simulink model "baseline1"  (R2022b)
settings: Solver=ode4  StartTime=0.0  StopTime=200  FixedStep=1e-3  RelTol=1e-3
undefined symbols (not defined in the file or in its folder): A_do, B_do, c_uf, do_w, f_b, f_max, f_min, F_TOT_MAX, Fz_min, g, G_do, Gamma_mix, Ixx, Iyy, Izz, K_eta, K_omega, K_w, Ka1, Ka2, Ka3, Kgamma, Knu, Kp1, Kp2, Kp3, L, l_axis, l_gain, m, m_p, n_state_axis, p2_bias_acc, p2_h3_s0, p2_ic_do, p2_ic_eso, p2_ic_pos, p2_ic_vel, p2_nd_pos, p2_prm, p2_prm_h3, p2_prm_m3, p2_prm_n6, p2_prm_w, p2_seed_acc, p2_seed_gyro, p2_seed_pos, p2_tau_m, p2_trim_do, p2_trim_eso, p2_trim_ff_v, p2_Ts_att, p2_Ts_pos, p2_var_acc, p2_var_gyro, p2_var_pos, payload_amp, payload_inj_on, payload_K_ratio, payload_model ... (+18)
(part 2 of 3)

== matlab function baseline1/Disturbances/Payload_Pendulum/pend_out ==
  data: xp input; d_mf output; a_uav input; m_p input; L input; g input; payload_z_on input
function d_mf = payload_pendulum_output(xp, a_uav, m_p, L, g, payload_z_on)
%#codegen
%PAYLOAD_PENDULUM_OUTPUT  Luc cap truyen len UAV = nhieu tai d_mf.
%
%  Paste noi dung file nay vao mot khoi MATLAB Function RIENG.
%  Tach roi khoi payload_pendulum_derivative theo dung kieu ma model dang
%  dung cho DO (do_derivative / do_output) va ESO.
%
%  Luc cang cap, moi truc:
%     T = m_p*( g*cos(th) + L*thdot^2 + a*sin(th) )
%  Phan luc ngang len UAV:
%     d = T*sin(th)
%
%  KHOP VOI BASELINE.  Trong translational_dynamics:
%     m*nu_dot = F - m*g*e3 + d_mf + d_lf
%  nen d_mf la LUC, don vi N, he QUAN TINH.  Dung het - khong chia khoi
%  luong, khong doi frame, khong doi dau.
%
%  ----------------------------------------------------------------------
%  THE VERTICAL COMPONENT (payload_z_on) - Part 3.5 (TEST_PLAN_PROMPT.md)
%  ----------------------------------------------------------------------
%  The tether pulls the UAV DOWN with force T*cos(th). At hover (th ~ 0),
%  T ~ m_p*g, so this pull is the payload's static weight - and it belongs
%  in the trim, not out of it: translational_dynamics.m's own equilibrium
%  (nu_dot = 0) gives F_act(3) = m*g - d_mf(3), so d_mf(3) = -T*cos(th)
%  makes the controller command F_act(3) = m*g + T ~ (m + m_p)*g at hover -
%  exactly the physical thrust margin table above, and exactly what
%  Checkpoint 3.5 measures.
%
%  An EARLIER version of this block computed d_z = m_p*g - T*cos(th_eff)
%  instead - subtracting the payload's own weight back out, so d_z ~ 0 at
%  hover and the trim point stayed IDENTICAL to m*g with no payload at all.
%  That was deliberate at the time (docs/devlog/AUDIT.md item 11 names it a
%  documented limitation, not an oversight): payload_z_on was reserved for a
%  future ablation and had never been turned on for any locked result, so
%  nothing published depended on its old behaviour. Checkpoint 3.5 is that
%  future ablation, and it explicitly requires the opposite: the payload's
%  weight DOES have to move the trim point, or "total thrust = (m + m_p)*g"
%  cannot be measured at all. Removing the +m_p*g cancellation term is the
%  whole fix.
%
%  payload_z_on = 0  (DEFAULT, unchanged - Stage 2.1's own bit-exact gate)
%     d_mf(3) = 0, identical to the original baseline (d_mf was horizontal
%     only). Only ONE thing differs between payload_model = 0 and 1: the
%     horizontal disturbance waveform. One experiment, one variable.
%  payload_z_on = 1
%     Adds the FULL vertical reaction, constant term included. Hover, no
%     wind: position stable, no saturation, total thrust = (m + m_p)*g
%     within 1% (Checkpoint 3.5) - not the near-zero-mean oscillation the
%     earlier version produced.

d_mf = zeros(3,1);

th_x = xp(1);  thd_x = xp(2);
th_y = xp(3);  thd_y = xp(4);

T_x = m_p*( g*cos(th_x) + L*thd_x^2 + a_uav(1)*sin(th_x) );
T_y = m_p*( g*cos(th_y) + L*thd_y^2 + a_uav(2)*sin(th_y) );

d_mf(1) = T_x*sin(th_x);
d_mf(2) = T_y*sin(th_y);

if payload_z_on > 0.5
    % Combined swing angle, used to project the tether tension onto z.
    th_eff  = sqrt(th_x^2 + th_y^2);
    T_eff   = m_p*( g*cos(th_eff) + L*(thd_x^2 + thd_y^2) );
    % Full reaction, including its constant (trim-shifting) part - see the
    % header. NOT m_p*g - T_eff*cos(th_eff): that cancelled the constant
    % term back out, which is exactly what Checkpoint 3.5 says must not
    % happen anymore.
    d_mf(3) = -T_eff*cos(th_eff);
end
end

== matlab function baseline1/Position_Observers/Payload_Predictor/pred_fcn ==
  data: gamma input; dmf_hat_p output; nu input; z input; l_gain input; do_w input; n_state_axis input; tau_pred input
function dmf_hat_p = payload_predictor(gamma, nu, z, l_gain, do_w, n_state_axis, tau_pred)
%#codegen
%PAYLOAD_PREDICTOR  Physical predictor for the payload disturbance: dmf_hat(t + tau).
%
%  Inputs
%     gamma, nu     : UAV position / velocity, inertial frame
%     z             : disturbance observer (DO) state, FLAT across all 3 axes
%     l_gain        : the DO's l gain (same as the DO_Out block)
%     do_w          : each exosystem block's frequency, FLAT across all 3
%                     axes, in the SAME order build_do_matrices.m used to
%                     build z (axis 1 in full, then axis 2, then axis 3)
%     n_state_axis  : 3x1, the number of STATES (not frequencies) each
%                     axis owns within z/xi_hat - Part 3.3 (TEST_PLAN_PROMPT.md)
%     tau_pred      : prediction horizon, s
%  Output
%     dmf_hat_p : the payload disturbance estimate AT TIME t + tau_pred, 3x1, N
%
%  ----------------------------------------------------------------------
%  PART 3.3: WHY n_state_axis WAS ADDED INSTEAD OF MAKING do_w A CELL
%  ----------------------------------------------------------------------
%  build/build_do_matrices.m's new form takes do_w_axis, a CELL {wx,wy,wz}
%  - but this is a %#codegen Simulink MATLAB Function block, and every
%  signal crossing a Simulink wire needs a FIXED SIZE at compile time;
%  Simulink cannot carry a cell type across a signal line. do_w here STAYS
%  a FLAT vector (exactly as before), just no longer IMPLICITLY split into
%  three equal shares - n_state_axis(i) says EXACTLY how many STATES (not
%  how many do_w entries) belong to axis i, and this function works out
%  how many do_w entries that is by accumulating block sizes (1 for DC, 2
%  for a harmonic) until that target is reached - the same logic
%  build_do_matrices.m uses to turn do_w_axis{i} into states, run in
%  reverse here.
%
%  With n_state_axis = [n_as;n_as;n_as] (all three axes equal, the
%  original case) and do_w in the OLD order, the loop below consumes
%  exactly n_as states per axis, identical to the old behaviour - which is
%  why Checkpoint 3.3's bit-exact gate (circle) needs no special-case branch.
%
%  ----------------------------------------------------------------------
%  DERIVATION (unchanged)
%  ----------------------------------------------------------------------
%  DO gia thiet nhieu tai sinh boi mot exosystem tuyen tinh, pt. (6):
%       xi_dot = A*xi,      d_mf = B*xi
%  Neu gia thiet do dung thi trang thai tuong lai biet duoc chinh xac:
%       xi(t + tau) = e^{A*tau} * xi(t)
%  va uoc luong hien tai la xi_hat = z + l*[gamma; nu]  (pt. 11a). Nen:
%       dmf_hat_p = B * e^{A*tau} * xi_hat
%
%  A la khoi cheo cac khoi 2x2 [0 w; -w 0], moi khoi mot tan so. e^{A*tau}
%  vi vay la mot phep QUAY, va MOI KHOI QUAY MOT GOC KHAC NHAU: khoi o tan so
%  w quay goc w*tau.
%       e^{A_k*tau} = [ cos(w_k*tau)   sin(w_k*tau);
%                      -sin(w_k*tau)   cos(w_k*tau) ]
%  Khong can expm - hai ham luong giac cho moi khoi.
%
%  B lay thanh phan LE cua moi khoi va CONG chung lai (d_mf cua mot truc la
%  tong dong gop cua cac hoa), nen chi can hang thu nhat cua moi phep quay:
%       dmf_hat_p(i) = sum_k [ cos(w_k*tau)*xi(le_k) + sin(w_k*tau)*xi(chan_k) ]
%
%  ----------------------------------------------------------------------
%  STATE ORDER - must match build_do_matrices
%  ----------------------------------------------------------------------
%  By AXIS first, then by FREQUENCY (in the order do_w_axis{i} lists them):
%       [axis1_freq1(1 or 2), axis1_freq2(...), axis2_freq1(...), ...]
%  With n_state_axis equal across axes and do_w in the old order, this
%  reduces to exactly the original 6/9/... state layout.
%
%  BLOCKS OF DIFFERENT SIZES, NOW ALSO ACROSS AXES (new - Part 3.3):
%  frequency 0 is the ONE-DIMENSIONAL DC mode, 1 state (§0.68 - 97.8% of
%  the payload channel's model error is a constant force); any other
%  frequency takes 2. The original code ASSUMED all 3 axes had the SAME
%  state count (numel(z) == 3*n_as); this one no longer does -
%  n_state_axis states it separately per axis.
%
%  ----------------------------------------------------------------------
%  TAU_PRED (unchanged)
%  ----------------------------------------------------------------------
%  Bang do tre HIEU DUNG tren duong luc, DO DUOC chu khong tinh ra: quet tau
%  o nhanh sin cho thay diem triet tieu (RMS_y = RMS_x) o tau = 140 ms.
%  Mo hinh chi tinh vong tu the bac hai cho 93 ms, nen ~47 ms den tu phan mo
%  hinh do khong co (phi tuyen thrust_attitude_ref, quan sat tu the, C(eta)).
%  Xem docs/AUDIT.md muc E.
%
%  ----------------------------------------------------------------------
%  GIOI HAN - PHAI GHI TRONG PAPER (khong doi)
%  ----------------------------------------------------------------------
%  Phep quay lay ca thanh phan CHAN cua exosystem vao dau ra. Thanh phan do
%  khong duoc quan sat truc tiep (B chi lay thanh phan le) nen sai so uoc
%  luong cua no lon hon, va bo du doan khuech dai no len theo sin(w*tau).
%  Do duoc: residual cua nhanh sin tang tu 0.0024 N (tau = 0) len 0.0118 N
%  (tau = 140 ms), voi mot vach moi hien ra dung o tan so sigma.
%  Do la mot gioi han tren THAT cho viec tang tau, khong phai loi cai dat.

dmf_hat_p = zeros(3,1);

xi_hat = z + l_gain*[gamma; nu];        % pt. (11a), giong DO_Out

% *** LOCK DIMENSIONS, per-axis version. ***
% If n_state_axis(i) does not match z's real state count, this fails
% SILENTLY in exactly the way the original warning described: the block
% keeps running, still outputs three plausible-looking numbers, just
% picking up the wrong axis's states. The assert below is the only guard.
assert(numel(n_state_axis) == 3, ...
    'payload_predictor: n_state_axis must have 3 elements.');
assert(sum(n_state_axis) == numel(z), ...
    ['payload_predictor: n_state_axis sums to %d, which does not match ' ...
     'z''s state count (%d). The Constant block feeding n_state_axis or ' ...
     'do_w is pointing at the wrong variable - re-run build_payload_predictor.'], ...
    sum(n_state_axis), numel(z));

n_w = numel(do_w);
b  = 0;   % state pointer (into z / xi_hat)
kw = 0;   % frequency pointer (into do_w)
for i = 1:3
    acc = 0;
    consumed = 0;
    while consumed < n_state_axis(i)
        kw = kw + 1;
        assert(kw <= n_w, ...
            'payload_predictor: ran out of do_w before axis %d had enough states.', i);
        w = do_w(kw);
        if w == 0
            % e^{0*tau} = 1: a constant predicts itself. This is why this
            % mode can never "predict wrong" - it only needs to be ESTIMATED.
            acc = acc + xi_hat(b+1);
            b = b + 1;
            consumed = consumed + 1;
        else
            c = cos(w*tau_pred);
            s = sin(w*tau_pred);
            acc = acc + c*xi_hat(b+1) + s*xi_hat(b+2);
            b = b + 2;
            consumed = consumed + 2;
        end
    end
    dmf_hat_p(i) = acc;
end
end

== matlab function baseline1/Position_Observers/IM_Est_Online/IM_Estimator ==
  data: vx input; w_hat_x output; vy input; t input; trust_x output; w_hat_y output; trust_y output; w_all_x output; mag_all_x output; w_all_y output; mag_all_y output
function [w_hat_x, trust_x, w_hat_y, trust_y, ...
          w_all_x, mag_all_x, w_all_y, mag_all_y] = im_est_estimator(vx, vy, t)
%#codegen
%IM_EST_ESTIMATOR  Online AR(2n) RLS + eig-based root-finding + Nyquist/
%  DC exclusion + per-slot nearest-neighbour assignment + trust gate +
%  coasting (docs/REGISTER_C.md sec 4.29/4.35/4.47). A codegen MATLAB
%  Function (Stateflow/EML) block - the SAME proven block type
%  Position_Observers/DO_12 (do_derivative) and Payload_Predictor
%  (payload_predictor) already use in this repo, not the legacy
%  Interpreted MATLAB Function block (multi-port support for that one
%  could not be verified without a MATLAB session to test against).
%  persistent state is standard, documented MATLAB Coder/Embedded
%  MATLAB practice. Every array here is FIXED SIZE (order=8 slots,
%  NaN-padded past the real count) - no dynamically-growing arrays, no
%  logical-index compaction, no nested structs - specifically to avoid
%  the variable-size codegen uncertainty that motivated (and then
%  un-motivated, sec 4.47) earlier design changes. Runs at fs=1Hz,
%  inherited from its input's sample time (the upstream Zero-Order
%  Hold in production; a From Workspace block at checkpoint 1.5).
%
%  Mirrors core/im_est_rls.m's own RLS update EXACTLY - same phi
%  convention (phi = -[x(k-1)..x(k-order)]), same lambda/order -
%  incrementally rather than in a batch loop, specifically so
%  checkpoint 1.5's 1e-9 rad/s agreement against that already-trusted
%  offline computation is a real regression test, not a coincidence.
%
%  Root-finding uses eig() of the companion matrix, not roots() -
%  roots() itself builds this same companion matrix internally and
%  calls eig() on it, so the values are identical by construction.
%
%  Untrusted slots (docs/REGISTER_C.md sec 4.29/4.35): |z|>=0.97 AND
%  <5% drift over the trailing 10 s AND t>=15s (a global floor, not a
%  per-slot "time since first trusted"). w_hat reports the 0.3 rad/s
%  placeholder for an untrusted slot - the internal tracking state is
%  NOT overwritten to the placeholder, so a slowly-converging slot
%  keeps its own continuity rather than being reset every untrusted
%  tick.
%
%  w_all_x/mag_all_x/w_all_y/mag_all_y (DIAGNOSTIC ONLY, sec 4.47
%  checkpoint 1.5): the raw ORDER=8 root set, BEFORE Nyquist/DC_GUARD
%  filtering or merging - directly comparable, element set for element
%  set (sort before comparing), to core/im_est_rls.m's own
%  R.roots(k,:) on identical input. Left unwired in the production
%  embedding - kept in this one file rather than forked into a second
%  copy, so the tested code and the deployed code never drift apart.

N_PAIRS = 4;
ORDER = 8;                      % 2*N_PAIRS, written as a literal for
                                 % codegen's fixed-size inference
LAM = 0.99;
NYQ_CUT = 0.9*pi;                % 0.9*Nyquist at DT_D = 1.0 s
DC_GUARD = 0.02;
DOMEGA_MIN = 0.05;
PLACEHOLDER = 0.3;
DRIFT_WIN = 10;
DRIFT_TOL = 0.05;
T_FLOOR = 15;

persistent theta_x theta_y P_x P_y buf_x buf_y n_seen_x n_seen_y
persistent slot_w_x slot_w_y slot_hist_x slot_hist_y

if isempty(n_seen_x)
    theta_x = zeros(ORDER,1); theta_y = zeros(ORDER,1);
    P_x = eye(ORDER)*1e3;     P_y = eye(ORDER)*1e3;
    buf_x = zeros(1,ORDER);   buf_y = zeros(1,ORDER);
    n_seen_x = 0;             n_seen_y = 0;
    slot_w_x = PLACEHOLDER*ones(1,N_PAIRS);
    slot_w_y = PLACEHOLDER*ones(1,N_PAIRS);
    slot_hist_x = PLACEHOLDER*ones(DRIFT_WIN,N_PAIRS);
    slot_hist_y = PLACEHOLDER*ones(DRIFT_WIN,N_PAIRS);
end

[theta_x, P_x, buf_x, n_seen_x, slot_w_x, slot_hist_x, w_hat_x, trust_x, w_all_x, mag_all_x] = ...
    tick_axis(theta_x, P_x, buf_x, n_seen_x, slot_w_x, slot_hist_x, vx, t, ...
    ORDER, N_PAIRS, LAM, NYQ_CUT, DC_GUARD, DOMEGA_MIN, PLACEHOLDER, DRIFT_TOL, T_FLOOR);
[theta_y, P_y, buf_y, n_seen_y, slot_w_y, slot_hist_y, w_hat_y, trust_y, w_all_y, mag_all_y] = ...
    tick_axis(theta_y, P_y, buf_y, n_seen_y, slot_w_y, slot_hist_y, vy, t, ...
    ORDER, N_PAIRS, LAM, NYQ_CUT, DC_GUARD, DOMEGA_MIN, PLACEHOLDER, DRIFT_TOL, T_FLOOR);
end

%% =====================================================================
function [theta, P, buf, n_seen, slot_w, slot_hist, w_hat, trust, w_all, mag_all] = ...
    tick_axis(theta, P, buf, n_seen, slot_w, slot_hist, v, t, order, n_pairs, ...
    lam, nyq_cut, dc_guard, domega_min, placeholder, drift_tol, t_floor)

% ---- RLS update (core/im_est_rls.m's own equations, incremental) ----
n_seen = n_seen + 1;
if n_seen > order
    phi   = -buf(:);
    e     = v - phi.'*theta;
    Pphi  = P*phi;
    denom = lam + phi.'*Pphi;
    Kk    = Pphi/denom;
    theta = theta + Kk*e;
    P     = (P - Kk*(Pphi.'))/lam;
end
buf = [v, buf(1:end-1)];

% ---- root-finding: companion matrix, eig() ----
c = theta(:).';
C = zeros(order,order);
C(1,:) = -c;
C(2:order,1:order-1) = eye(order-1);
r = eig(C);

w_all = abs(angle(r)).';          % 1 x order, DT_D = 1.0 s
mag_all = abs(r).';               % 1 x order

% ---- Nyquist/DC_GUARD exclusion + close-frequency merge, FIXED SIZE
% (order slots, NaN = not present) - no dynamically-growing arrays ----
w_cand = nan(1,order); m_cand = nan(1,order);
keep = (w_all <= nyq_cut) & (w_all > dc_guard);
w_tmp = w_all; w_tmp(~keep) = NaN;
m_tmp = mag_all; m_tmp(~keep) = NaN;
[w_tmp_sorted, ord] = sort(w_tmp);           % NaNs sort to the end
m_tmp_sorted = m_tmp(ord);
n_cand = 0;
for i = 1:order
    if isnan(w_tmp_sorted(i)), continue; end
    if n_cand > 0 && (w_tmp_sorted(i) - w_cand(n_cand) < domega_min)
        if m_tmp_sorted(i) > m_cand(n_cand)
            w_cand(n_cand) = w_tmp_sorted(i);
            m_cand(n_cand) = m_tmp_sorted(i);
        end
    else
        n_cand = n_cand + 1;
        w_cand(n_cand) = w_tmp_sorted(i);
        m_cand(n_cand) = m_tmp_sorted(i);
    end
end

% ---- greedy nearest-neighbour slot assignment (sec 4.29 item 4a);
% unmatched slots COAST - slot_w stays at its previous value. Fixed
% size throughout: n_pairs slots, order candidate cells (only the
% first n_cand are ever valid, the rest are NaN and never selected). ----
assigned = false(1,n_pairs);
mag_assigned = zeros(1,n_pairs);
avail = ~isnan(w_cand);
for pass = 1:n_pairs
    bestSlot = 0; bestCand = 0; bestDist = Inf;
    for s = 1:n_pairs
        if assigned(s), continue; end
        for k = 1:order
            if ~avail(k), continue; end
            d = abs(w_cand(k) - slot_w(s));
            if d < bestDist
                bestDist = d; bestSlot = s; bestCand = k;
            end
        end
    end
    if bestSlot == 0, break; end
    slot_w(bestSlot) = w_cand(bestCand);
    mag_assigned(bestSlot) = m_cand(bestCand);
    assigned(bestSlot) = true;
    avail(bestCand) = false;
end

slot_hist = [slot_hist(2:end,:); slot_w];

trust = false(1,n_pairs);
for s = 1:n_pairs
    h  = slot_hist(:,s);
    mh = mean(h);
    drift = (max(h)-min(h)) / max(mh, eps);
    trust(s) = assigned(s) && (mag_assigned(s) >= 0.97) && ...
               (drift < drift_tol) && (t >= t_floor);
end

w_hat = slot_w;
w_hat(~trust) = placeholder;
end

== matlab function baseline1/Position_Observers/IM_Est_Online/IM_Rebuild ==
  data: w_hat_x input; A_do output; trust_x input; w_hat_y input; trust_y input; wn_p input; sigma_z input; l_axis input; strict input; B_do output; l_gain output; G_do output; fallback output; reason output
function [A_do, B_do, l_gain, G_do, fallback, reason] = ...
    im_est_do_rebuild(w_hat_x, trust_x, w_hat_y, trust_y, wn_p, sigma_z, l_axis, strict)
%#codegen
%IM_EST_DO_REBUILD  Online IM = {0, w_hat_k, wn_p} internal-model
%  matrix rebuild (docs/REGISTER_C.md sec 4.29/4.35/4.46/4.47) - a
%  codegen MATLAB Function (Stateflow/EML) block, the SAME proven
%  block type as im_est_estimator.m and do_derivative/
%  payload_predictor, not build_do_matrices.m called directly:
%  build_do_matrices.m's cell-array/varargin dispatch is not verified
%  codegen-safe, and this function's do_w_axis STRUCTURE never varies
%  (always DC + 4 harmonics + wn_p on x/y, the unchanged {0,sigma_z}
%  on z - n_state = 25, fixed) - only the FREQUENCY VALUES at each
%  slot change - so a direct, fixed-index construction is used
%  instead, with build_do_matrices.m's own stability check (eig(A_cl)
%  < 0) replicated exactly. The CONSTRUCTION-EQUIVALENCE checkpoint
%  (sec 4.47) - forcing every slot to the exact-frequency reference's
%  own values and comparing against build_do_matrices's OWN output
%  bit for bit - exists specifically to catch a construction error
%  here, so drift is not asserted away, it is tested for.
%
%  State order (sec 4.46's own fixed layout, matching
%  build_do_matrices.m's "by axis first, then by frequency" rule with
%  the harmonics in slot order 1-4, then wn_p):
%    x: [1]=DC [2 3]=h1 [4 5]=h2 [6 7]=h3 [8 9]=h4 [10 11]=wn_p
%    y: [12]=DC [13 14]=h1 [15 16]=h2 [17 18]=h3 [19 20]=h4 [21 22]=wn_p
%    z: [23]=DC [24 25]=sigma_z
%
%  DECOUPLING (sec 4.47 item 3, the refinement to sec 4.29/4.35's
%  placeholder-only design): an untrusted harmonic slot (trust_x/y(k)
%  false) still occupies its 2 states (fixed size, sec 4.47's own
%  registered reasoning) but gets l_gain=0 for both AND is excluded
%  from B_do - completely inert, not merely mistuned. DC and wn_p are
%  never coasted/untrusted, so decoupling only ever applies to the 4
%  harmonic slots per axis.
%
%  FALLBACK (sec 4.46 item 1): candidate frequencies within
%  DOMEGA_MIN=0.05 rad/s of each other (checked among the axis's own
%  4 harmonics + wn_p - a defensive check on the REBUILD input, in
%  addition to im_est_estimator.m's own pre-assignment merge, sec
%  4.47's own note) OR a resulting UNSTABLE Acl -> HOLD the previous
%  A_do/B_do/l_gain (persistent, fixed-size - no Memory-block feedback
%  needed, same reasoning as im_est_estimator.m's own state) and
%  report fallback=true, reason (1=dup, 2=unstable). strict=true skips
%  the hold and errors immediately instead - for checkpoint-building
%  only, never a production/scored run (sec 4.46 item 1c).

N = 25;
DOMEGA_MIN = 0.05;
M_UAV = 1.121;

persistent A_prev B_prev L_prev initialized
if isempty(initialized)
    A_prev = zeros(N,N);
    B_prev = zeros(3,N);
    L_prev = zeros(N,6);
    initialized = true;
end

G_do = (1/M_UAV)*[zeros(3,3); eye(3)];

% ---- defensive dup check: each axis's own 4 harmonics + wn_p ----
% Only TRUSTED harmonics (+ wn_p, always trusted) can collide in a way
% that matters: a decoupled/untrusted slot is excluded from B_do and
% l_gain, so its frequency value never enters Acl's own observable
% dynamics - two untrusted slots sharing the SAME placeholder (as every
% slot does before any is trusted, during warmup) is not a real
% duplicate in the sense build_do_matrices.m's own assertion guards
% against, and must not spuriously trigger a fallback.
tx = [trust_x(1) trust_x(2) trust_x(3) trust_x(4) true];
dup = false;
fx = [w_hat_x(1) w_hat_x(2) w_hat_x(3) w_hat_x(4) wn_p];
for i = 1:5
    for j = i+1:5
        if tx(i) && tx(j) && abs(fx(i)-fx(j)) < DOMEGA_MIN, dup = true; end
    end
end
ty = [trust_y(1) trust_y(2) trust_y(3) trust_y(4) true];
fy = [w_hat_y(1) w_hat_y(2) w_hat_y(3) w_hat_y(4) wn_p];
for i = 1:5
    for j = i+1:5
        if ty(i) && ty(j) && abs(fy(i)-fy(j)) < DOMEGA_MIN, dup = true; end
    end
end

if dup && strict
    error('im_est_do_rebuild:dup', 'candidate frequencies within DOMEGA_MIN of each other (strict mode).');
end

A_new = zeros(N,N);
B_new = zeros(3,N);
L_new = zeros(N,6);

% ---- x axis: states 1..11 ----
A_new(1,1) = 0;  B_new(1,1) = 1;  L_new(1,4) = l_axis(1);
[A_new, B_new, L_new] = put_harm(A_new, B_new, L_new, 2, w_hat_x(1), l_axis(1), 1, trust_x(1));
[A_new, B_new, L_new] = put_harm(A_new, B_new, L_new, 4, w_hat_x(2), l_axis(1), 1, trust_x(2));
[A_new, B_new, L_new] = put_harm(A_new, B_new, L_new, 6, w_hat_x(3), l_axis(1), 1, trust_x(3));
[A_new, B_new, L_new] = put_harm(A_new, B_new, L_new, 8, w_hat_x(4), l_axis(1), 1, trust_x(4));
[A_new, B_new, L_new] = put_harm(A_new, B_new, L_new, 10, wn_p, l_axis(1), 1, true);

% ---- y axis: states 12..22 ----
A_new(12,12) = 0;  B_new(2,12) = 1;  L_new(12,5) = l_axis(2);
[A_new, B_new, L_new] = put_harm(A_new, B_new, L_new, 13, w_hat_y(1), l_axis(2), 2, trust_y(1));
[A_new, B_new, L_new] = put_harm(A_new, B_new, L_new, 15, w_hat_y(2), l_axis(2), 2, trust_y(2));
[A_new, B_new, L_new] = put_harm(A_new, B_new, L_new, 17, w_hat_y(3), l_axis(2), 2, trust_y(3));
[A_new, B_new, L_new] = put_harm(A_new, B_new, L_new, 19, w_hat_y(4), l_axis(2), 2, trust_y(4));
[A_new, B_new, L_new] = put_harm(A_new, B_new, L_new, 21, wn_p, l_axis(2), 2, true);

% ---- z axis: states 23..25 (unchanged {0, sigma_z} - never estimated) ----
A_new(23,23) = 0;  B_new(3,23) = 1;  L_new(23,6) = l_axis(3);
[A_new, B_new, L_new] = put_harm(A_new, B_new, L_new, 24, sigma_z, l_axis(3), 3, true);

% ---- stability check on the ACTIVE subsystem only ----
% A decoupled harmonic block still carries its own [0 w;-w 0] open-loop
% dynamics in A_new (by design - sec 4.47 item 3: the state exists and
% evolves, just isolated), whose eigenvalues sit exactly on the
% imaginary axis (Re=0) - marginally stable, not Re<0. Checking eig()
% of the FULL Acl would fail this test whenever ANY slot is untrusted,
% including the entire warmup period before t>=15s, which defeats the
% design (constant spurious fallback). Since a decoupled block is
% provably block-diagonal (B_new/L_new are both zero for it - no
% coupling in or out), its own marginal eigenvalues are harmless and
% irrelevant to whether the ACTIVE subsystem is stable. A_check patches
% each decoupled block's diagonal to a trivially-stable dummy (-I),
% fixed-index (no variable-size extraction needed) - it changes nothing
% about the ACTUAL A_do returned below, only what stability is
% evaluated against.
A_check = A_new;
A_check = patch_if_untrusted(A_check, 2,  trust_x(1));
A_check = patch_if_untrusted(A_check, 4,  trust_x(2));
A_check = patch_if_untrusted(A_check, 6,  trust_x(3));
A_check = patch_if_untrusted(A_check, 8,  trust_x(4));
A_check = patch_if_untrusted(A_check, 13, trust_y(1));
A_check = patch_if_untrusted(A_check, 15, trust_y(2));
A_check = patch_if_untrusted(A_check, 17, trust_y(3));
A_check = patch_if_untrusted(A_check, 19, trust_y(4));

Acl = A_check - L_new*G_do*B_new;
ev = eig(Acl);
stable = max(real(ev)) < 0;

if (~stable) && strict
    error('im_est_do_rebuild:unstable', 'Acl not stable with the current w_hat (strict mode).');
end

if dup || ~stable
    A_do = A_prev; B_do = B_prev; l_gain = L_prev;
    fallback = true;
    if dup, reason = 1; else, reason = 2; end
else
    A_do = A_new; B_do = B_new; l_gain = L_new;
    A_prev = A_new; B_prev = B_new; L_prev = L_new;
    fallback = false;
    reason = 0;
end
end

%% =====================================================================
function [A, B, L] = put_harm(A, B, L, idx1, w, lg, axis_col, trust)
%PUT_HARM  Place one 2-state harmonic block at states idx1,idx1+1 -
%  build_do_matrices.m's own [0 w;-w 0] / B_do(i,b+1)=1 / l_gain
%  pattern, fixed-index. trust=false -> decoupled (sec 4.47 item 3):
%  l_gain stays 0 for both states, B stays 0 - the state still exists
%  (fixed size) but contributes to and is corrected by nothing.
idx2 = idx1 + 1;
A(idx1,idx1) = 0;  A(idx1,idx2) = w;
A(idx2,idx1) = -w; A(idx2,idx2) = 0;
if trust
    B(axis_col, idx1) = 1;
    L(idx1, 3+axis_col) = lg;
    L(idx2, 3+axis_col) = lg;
end
end

%% =====================================================================
function A = patch_if_untrusted(A, idx1, trust)
%PATCH_IF_UNTRUSTED  For the stability check only (sec 4.47's own
%  reasoning, see the caller): a decoupled block's marginal (Re=0)
%  open-loop eigenvalues are harmless (B/l_gain are already zero for
%  it, so it cannot destabilize anything, block-diagonal) but would
%  otherwise fail max(real(eig(.)))<0 spuriously. Overwrite ONLY the
%  stability-check copy's diagonal block to a trivially-stable dummy.
if ~trust
    idx2 = idx1 + 1;
    A(idx1,idx1) = -1; A(idx1,idx2) = 0;
    A(idx2,idx1) = 0;  A(idx2,idx2) = -1;
end
end

== matlab function baseline1/P2/P2_Core/P2/P2_Trans ==
  data: x input double size=[12 1]; dx output double size=[12 1]; f_act input double size=1; eta input double size=[3 1]; w input double size=[3 1]; prm input double size=[8 1]; gam output double size=[3 1]; nu output double size=[3 1]; a_Q output double size=[3 1]; d_mf output double size=[3 1]; d_lf output double size=[3 1]; mon output double size=[5 1]
function [dx, gam, nu, a_Q, d_mf, d_lf, mon] = p2_trans(x, f_act, eta, w, prm)
%#codegen
%P2_TRANS  MATLAB Function block P2/P2_Core/P2/P2_Trans (GD2b, plant_model = 1).
%
%  Translational dynamics of the UAV + 3-D rigid-cable pendulum of plant P2. The
%  equations are NOT written here: this block calls core/plant_p2_free.m, the same
%  code verified offline by verification/verify_plant_p2.m (GD2a, 41/41).
%
%  In   x      12x1 state [x_Q; v_Q; q; omega] (Integrator P2_x, IC p2_x0)
%       f_act  total thrust AFTER the motor lag [N] (Gamma_mix * f, row 1)
%       eta    TRUE Euler angles (tag eta, Int_eta)
%       w      3x1 true wind [m/s]; the vertical component is dropped here (spec sec 5)
%       prm    [m_Q; m_L; L; g; zeta_s; K; K_w; U_ref]   (p2_prm, core/p2_setup.m)
%  Out  dx     12x1 state derivative
%       gam, nu, a_Q   true position, velocity, acceleration of the UAV
%       d_mf   T q - F_d  (cable force on the UAV, for logging)
%       d_lf   F_wQ       (wind force on the body, for logging)
%       mon    [T; slack; ||q|-1|; |omega.q|; theta]  (REGISTER_P2 sec 0.4 flags)

% Output sizes declared first (as every v1 block does, e.g. xp_dot = zeros(4,1)):
% the block sits in a loop with Integrator P2_x, and Simulink must know the output
% sizes before it knows the input sizes (GD2b, second build attempt).
dx   = zeros(12, 1);
gam  = zeros(3, 1);
nu   = zeros(3, 1);
a_Q  = zeros(3, 1);
d_mf = zeros(3, 1);
d_lf = zeros(3, 1);
mon  = zeros(5, 1);

P = struct('mode', 'free', 'g', prm(4), 'm_Q', prm(1), 'm_L', prm(2), 'L', prm(3), ...
           'zeta_s', prm(5), 'K', prm(6), 'K_w', prm(7), 'U_ref', prm(8));
F = force_from_attitude(f_act, eta);
[dx, o] = plant_p2_free(x, F, [w(1); w(2); 0], P);
gam  = x(1:3);
nu   = x(4:6);
a_Q  = dx(4:6);
d_mf = o.d_mf;
d_lf = o.d_lf;
qh   = x(7:9) / norm(x(7:9));
mon  = [o.T; double(o.slack); o.qnorm_err; o.wq; acos(max(min(-qh(3), 1), -1))];
end

== matlab function baseline1/P2/P2_Core/P2/P2_WindHat ==
  data: w input double size=[3 1]; dlf_hat output double size=[3 1]; nu_c input double size=[3 1]; prm_w input double size=[2 1]
function dlf_hat = p2_wind_force_hat(w, nu_c, prm_w)
%#codegen
%P2_WIND_FORCE_HAT  MATLAB Function block P2/P2_Core/P2/P2_WindHat (GD2b, plant_model = 1).
%
%  The controller's wind-force model on P2 (REGISTER_P2 sec 0.3): quadratic, the same
%  form as the plant's body drag, NOMINAL parameters, relative velocity w - v_Q with
%  the controller's own MEASURED velocity nu_c:
%     dlf_hat = (K_w/U_ref) |w - nu_c| (w - nu_c)
%  w is the SELECTED wind (sensor / PI-MoE / oracle, as WSEL); vertical component dropped.
%  prm_w = [K_w; U_ref]. Replaces K_w*w (WM_Kw / WP_Kw / WO_Kw) only when plant_model = 1.

dlf_hat = zeros(3, 1);          % output size declared first, as every v1 block does
r = [w(1); w(2); 0] - nu_c;
dlf_hat = (prm_w(1) / prm_w(2)) * norm(r) * r;
end

== matlab function baseline1/P2/P2_Core/P2/P2_N6 ==
  data: s input double size=[4 1]; s_next output double size=[4 1]; w_meas input double size=[3 1]; w_sig input double size=[3 1]; vQ input double size=[3 1]; dmf_do input double size=[3 1]; gate input double size=1; prm input double size=[17 1]; delta output double size=[3 1]; mon output double size=[5 1]
function [s_next, delta, mon] = p2_n6_term(s, w_meas, w_sig, vQ, dmf_do, gate, prm)
%#codegen
%P2_N6_TERM  MATLAB Function block P2/P2_Core/P2/P2_N6 (REGISTER_P2 sec 15.4, 18.2; N6).
%
%  Wind -> payload term added to the controller's payload channel (active only when
%  p2_n6 = 1; otherwise the block is not compiled). Runs at the base step h (inputs held).
%
%  In   s       4x1 observer state at t, [theta_x; theta_dot_x; theta_y; theta_dot_y]
%               (Unit Delay N6_s, IC 0)
%       w_meas  3x1 measured wind (the sensor, 50 ms late) - drives the observer in EVERY column
%       w_sig   3x1 the column's wind (as WSEL: sensor / PI-MoE / oracle) - held over the
%               horizon; the ONLY input that differs between the N6 columns
%       vQ      3x1 the controller's measured velocity nu_c
%       dmf_do  3x1 the DO's payload estimate (DO_Out, before the payload predictor)
%       gate    wind_pred_on * wvalid (as WD_gate): the term is applied only while the
%               controller uses its wind model at all
%       prm     17x1 core/p2_n6_prm.m
%  Out  s_next  4x1 state at t + h: s(k+1) = Phi_o s(k) + Gam_o [u; dmf_do_h / (m_L g)]
%       delta   3x1 added to the payload channel:
%               pend_lin_predict(s, w_sig, vQ) - m_L g theta(t)   (the predicted CHANGE of the
%               horizontal cable force over tau; the DO already carries the present force)
%       mon     5x1 [theta_x; theta_y; delta_x; delta_y; gate] (log)
s_next = zeros(4, 1);
delta  = zeros(3, 1);
mon    = zeros(5, 1);
Phi_o = reshape(prm(1:4), 2, 2);
Gam_o = reshape(prm(5:8), 2, 2);
C = prm(15);  kL = prm(16);  L = prm(17);
S = [s(1), s(3); s(2), s(4)];
% observer: u from the measured wind, relative velocity w - v_L, v_L = v_Q + L theta_dot
r = [w_meas(1) - vQ(1) - L * S(2, 1); w_meas(2) - vQ(2) - L * S(2, 2)];
u = kL * norm(r) * r;
for a = 1:2
    sa = Phi_o * S(:, a) + Gam_o * [u(a); dmf_do(a) / C];
    s_next(2 * a - 1) = sa(1);
    s_next(2 * a)     = sa(2);
end
% prediction tau ahead with the column's wind held
d_pred = pend_lin_predict(S, w_sig, vQ, prm(9:17));
if gate >= 0.5
    delta(1) = d_pred(1) - C * S(1, 1);
    delta(2) = d_pred(2) - C * S(1, 2);
end
mon = [S(1, 1); S(1, 2); delta(1); delta(2); gate];
end

== matlab function baseline1/P2/P2_Core/P2/P2_H3 ==
  data: s input double size=[7 1]; s_next output double size=[7 1]; a_meas input double size=[3 1]; f_cmd input double size=1; eta input double size=[3 1]; prm input double size=[11 1]; d_hat output double size=[3 1]
function [s_next, d_hat] = p2_h3_indi(s, a_meas, f_cmd, eta, prm)
%#codegen
%P2_H3_INDI  MATLAB Function block P2/P2_Core/P2/P2_H3 (REGISTER_P2 sec 40.1; competitor H3).
%
%  Acceleration-based disturbance estimate of the INDI type (outer loop of Smeur 2018) - NOT a
%  full INDI controller. Runs at the attitude rate (inputs held); read by the loop only through
%  the Variant P2_CMP_Sel (p2_cmp = 1: d_mf_hat := d_hat, d_lf_hat := 0).
%
%  In   s       7x1 state at t: [T; x_x(2); x_y(2); x_z(2)] (Unit Delay H3_s, IC below)
%       a_meas  3x1 the accelerometer (inertial frame, noise and bias as nominal)
%       f_cmd   total-thrust command [N] (fthr_c)
%       eta     3x1 the MEASURED attitude (eta_c)
%       prm     11x1 core/p2_h3_prm.m
%  Out  s_next  7x1 state at t + h
%       d_hat   3x1 H(z)[m a_meas - F_thr_hat + m g e3], F_thr_hat = force_from_attitude(T, eta)
s_next = zeros(7, 1);
d_hat  = zeros(3, 1);
Phi = reshape(prm(1:4), 2, 2);
Gam = prm(5:6);
Cf  = reshape(prm(7:8), 1, 2);
aT = prm(9);  m = prm(10);  g = prm(11);
T = s(1);
F = force_from_attitude(T, eta);
u = m * a_meas - F + m * g * [0; 0; 1];
s_next(1) = aT * T + (1 - aT) * f_cmd;
for a = 1:3
    x = s(2 * a:2 * a + 1);
    d_hat(a) = Cf * x;
    s_next(2 * a:2 * a + 1) = Phi * x + Gam * u(a);
end
end

== matlab function baseline1/P2/P2_Core/P2/P2_H3_out ==
  data: s input double size=[7 1]; d_hat output double size=[3 1]; prm input double size=[11 1]
function d_hat = p2_h3_out(s, prm)
%#codegen
%P2_H3_OUT  MATLAB Function block P2/P2_Core/P2/P2_H3_out (REGISTER_P2 sec 40.1, sec 50.5; competitor H3).
%
%  The H3 estimate read from the filter STATE only: d_hat(a) = Cf x_a, x_a = s(2a:2a+1) - the same
%  arithmetic as the d_hat output of p2_h3_indi.m. A MATLAB Function block is direct feedthrough on every
%  input, so taking d_hat from P2_H3 (which also reads the thrust command f_cmd) closed an algebraic loop
%  position law -> thrust -> P2_H3 -> dmf_hat -> position law at the first H3 build; this block reads only the
%  Unit Delay H3_s and the parameters, so the loop is broken and the values are unchanged.
%
%  In   s    7x1 state at t (Unit Delay H3_s)
%       prm  11x1 core/p2_h3_prm.m
%  Out  d_hat 3x1
d_hat = zeros(3, 1);
Cf = reshape(prm(7:8), 1, 2);
for a = 1:3
    x = s(2 * a:2 * a + 1);
    d_hat(a) = Cf * x;
end
end

== matlab function baseline1/P2/P2_Core/P2/P2_M3 ==
  data: s input double size=[4 1]; s_next output double size=[4 1]; w_meas input double size=[3 1]; vQ input double size=[3 1]; gam_d input double size=[3 1]; nu_d input double size=[3 1]; acc_d input double size=[3 1]; gam_c input double size=[3 1]; a_meas input double size=[3 1]; prm input double size=[30 1]; dM_now output double size=[3 1]; dM_pred output double size=[3 1]; mon output double size=[6 1]
function [s_next, dM_now, dM_pred, mon] = p2_m3_term(s, w_meas, vQ, gam_d, nu_d, acc_d, gam_c, a_meas, prm)
%#codegen
%P2_M3_TERM  MATLAB Function block P2/P2_Core/P2/P2_M3 (REGISTER_P2 sec 45; GD8 (iii) FULL).
%
%  Open-loop linear pendulum model of the payload force (no correction from any payload-state
%  estimate, sec 45.7). Runs at the base step h (inputs held). Read by the loop only when p2_m3 = 1
%  (Position_Observers: P2_M3_Sel adds dM_pred to the payload channel, P2_M3_DoSel adds dM_now to the
%  DO's known-input port); with p2_m3 = 0 nothing reads it (value-neutral).
%
%  In   s       4x1 model state at t, [theta_x; theta_dot_x; theta_y; theta_dot_y] (Unit Delay M3_s, IC 0 =
%               hanging at rest, like the plant)
%       w_meas  3x1 measured wind (the sensor, 50 ms late, 20 Hz hold); vertical dropped
%       vQ      3x1 the controller's measured velocity nu_c
%       gam_d, nu_d, acc_d   3x1 the reference (trajectory_ref)
%       gam_c   3x1 the controller's measured position gamma_c
%       a_meas  3x1 the accelerometer (read only when prm(28) = 1, (iii-m))
%       prm     30x1 core/p2_m3_prm.m
%  Out  s_next  4x1 state at t + h: s(k+1) = Phi_h s(k) + Gam_h [F_wL; a_c]
%       dM_now  3x1 the model's payload force at t:  [C theta_x; C theta_y; -m_L (g + a_c,z)]
%       dM_pred 3x1 the same tau_m ahead with the inputs held (exact ZOH)
%       mon     6x1 [theta_x; theta_y; dM_pred(1:3); a_c,z] (log)
%
%  a_c = a_d - g e3 with a_d of Guo (9) recomputed from the reference and the measured state:
%     a_d = Kgamma (gamma_d - gamma_c) + Knu (nu_d - nu_c) + g e3 + acc_d
%  (no estimate enters, so no algebraic loop; p2_setup refuses M3 with the LQI law on).
s_next  = zeros(4, 1);
dM_now  = zeros(3, 1);
dM_pred = zeros(3, 1);
mon     = zeros(6, 1);
Phi_h = reshape(prm(1:4), 2, 2);    Gam_h = reshape(prm(5:8), 2, 2);
Phi_t = reshape(prm(9:12), 2, 2);   Gam_t = reshape(prm(13:16), 2, 2);
C = prm(17);  kL = prm(18);  L = prm(19);  m_L = prm(20);  g = prm(21);
Kg = prm(22:24);  Kn = prm(25:27);  acc_meas = prm(28);
if acc_meas >= 0.5
    a_c = a_meas;
else
    a_c = Kg .* (gam_d - gam_c) + Kn .* (nu_d - vQ) + acc_d;     % = a_d - g e3
end
S = [s(1), s(3); s(2), s(4)];
% wind force on the payload: relative velocity w - v_L, v_L = v_Q + L theta_dot (horizontal, small angle)
r = [w_meas(1) - vQ(1) - L * S(2, 1); w_meas(2) - vQ(2) - L * S(2, 2)];
F = kL * norm(r) * r;
for a = 1:2
    u = [F(a); a_c(a)];
    sn = Phi_h * S(:, a) + Gam_h * u;
    sp = Phi_t * S(:, a) + Gam_t * u;
    s_next(2 * a - 1) = sn(1);
    s_next(2 * a)     = sn(2);
    dM_now(a)  = C * S(1, a);
    dM_pred(a) = C * sp(1);
end
dM_now(3)  = -m_L * (g + a_c(3));
dM_pred(3) = dM_now(3);
mon = [S(1, 1); S(1, 2); dM_pred; a_c(3)];
end

== matlab function baseline1/Trajectory/Traj_Ref ==
  data: t input; gamma_d output; R input; w input; z0 input; nu_d output; acc_d output; tau_prev input; traj_type input; traj_par input
function [gamma_d, nu_d, acc_d] = trajectory_ref(t, R, w, z0, tau_prev, traj_type, traj_par)
%#codegen
% --- Khai bao kich thuoc output (de Simulink suy dung kich thuoc tin hieu) ---
gamma_d = zeros(3,1); nu_d = zeros(3,1); acc_d = zeros(3,1);
%
% traj_type selects the horizontal path; z is always z0 (constant altitude).
%   0  hover        R forced to 0 - see the note at that case, below
%   1  circle       R, w as before (Test 2-4 of the reference work)
%   2  figure-8 (Gerono)   x = A sin(w t), y = (A/2) sin(2 w t)
%   3  square, min-jerk edges, side D, edge time T, dwell T_h at each corner
%   4  multi-sine, four fixed frequencies, fixed phases, one amplitude scale
%
% traj_par is a FIXED-SIZE 4x1 vector (codegen requires fixed size), read
% differently by each type - see the case bodies. Types that need nothing
% from it (hover, circle) ignore it entirely.
%
% TEST_PLAN_PROMPT.md's Part 3.1 specifies the standard params for each type
% (T3a/T3b for figure-8, etc.) and this file only implements the geometry; it
% chooses no numbers of its own. This is infrastructure, not a scored
% experiment - no docs/REGISTER_*.md covers it, because the campaign's own
% rule only requires one per lettered phase (A-E) that scores a prediction.
%
% ------------------------------------------------------------------
% tau_prev : REFERENCE PREVIEW (docs/REGISTER_TAU.md §A2). Unchanged by this
%            addition, and unchanged in scope: it applies to acc_d ONLY.
%            gamma_d and nu_d stay at t for every traj_type, for the same
%            reason as before - gamma_d is what Err_Norm measures error
%            against, and advancing it would move the target rather than
%            improve tracking of it.
%
%            For traj_type = 1 this is still literally a ROTATION of the
%            reference-acceleration vector, because a circle's acc_d is one
%            sinusoid. For every other type there is no single frequency to
%            rotate by, so the general form is used instead: acc_d is the
%            SAME closed-form function of time as gamma_d/nu_d, evaluated at
%            t + tau_prev rather than at t. At traj_type = 1 the general form
%            and the rotation are the same computation (cos/sin of w*(t+tau)),
%            so this is not a second implementation living beside the first -
%            it IS the first, generalised.
%
%            tau_prev = 0 must reproduce the un-previewed trajectory bit for
%            bit at every traj_type, because t + 0 == t exactly. That is
%            checkpoint 3.1's "no-disturbance, closed-loop RMS" gate reduced
%            to its open-loop half, and verification/traj_check.m checks it directly.
%
% ------------------------------------------------------------------
% CODEGEN NOTES
% ------------------------------------------------------------------
% No persistent state: every type is a pure function of t. mod() is a
% MATLAB Coder / Stateflow supported function; used only in case 3.
% traj_par is read positionally and never resized - MATLAB Function blocks
% require fixed-size signals, and a 4x1 in every branch keeps the port
% width the same regardless of which traj_type is selected at run time.

tp = t + tau_prev;

switch traj_type
case 0
    % Hover. Mathematically IDENTICAL to case 1 with R = 0 - cos(w*t)*0 = 0
    % regardless of t or w, so nothing about w matters here. Written as its
    % own branch anyway, rather than forcing R = 0 into case 1 from the
    % caller, because a caller that forgets to zero R would otherwise fly a
    % circle while believing it had selected hover. verification/traj_check.m
    % verifies the two branches agree exactly at R = 0, so there are not two
    % independent implementations of the same geometry, only one written
    % twice for safety - and the check that they match is what keeps that
    % true.
    gamma_d = [0; 0; z0];
    nu_d    = [0; 0; 0];
    acc_d   = [0; 0; 0];

case 1
    % Circle (baseline). UNCHANGED from the pre-existing file, to the
    % character: this is checkpoint 3.1's bit-exactness gate.
    gamma_d = [R*cos(w*t);       R*sin(w*t);       z0];
    nu_d    = [-R*w*sin(w*t);    R*w*cos(w*t);     0 ];
    acc_d   = [-R*w^2*cos(w*tp); -R*w^2*sin(w*tp); 0 ];

case 2
    % Figure-8 (Gerono). x = A sin(w t), y = (A/2) sin(2 w t).
    % traj_par(1) = A. w is the SAME input circle uses - T3a reuses circle's
    % w = 1.575 rad/s so the y-axis runs at 2w = 3.15 rad/s (deliberately
    % near the pendulum's natural frequency at L = 1.0, per the registration);
    % T3b uses w = 0.7875 rad/s, off resonance.
    A = traj_par(1);
    gamma_d = [ A*sin(w*t);              (A/2)*sin(2*w*t);              z0];
    nu_d    = [ A*w*cos(w*t);             A*w*cos(2*w*t);                0];
    acc_d   = [-A*w^2*sin(w*tp);        -2*A*w^2*sin(2*w*tp);            0];

case 3
    % Square, min-jerk edges. traj_par = [D; T; T_h; 0] - side length, edge
    % duration, corner dwell. A closed, counterclockwise square centred on
    % the origin (like the circle and the figure-8), corners at
    % (D/2,-D/2) -> (D/2,D/2) -> (-D/2,D/2) -> (-D/2,-D/2) -> back to start.
    D   = traj_par(1);
    T   = traj_par(2);
    T_h = traj_par(3);
    h   = D/2;
    CORNERS = [ h -h;  h h;  -h h;  -h -h ];   % 4x2, row k = corner k (0-based)
    [p, v, ~]  = square_minjerk(t,  CORNERS, T, T_h);
    [~, ~, ap] = square_minjerk(tp, CORNERS, T, T_h);
    gamma_d = [p(1); p(2); z0];
    nu_d    = [v(1); v(2); 0];
    acc_d   = [ap(1); ap(2); 0];

case 4
    % Multi-sine. Frequencies and phases are FIXED CONSTANTS, not run-time
    % inputs: a reference trajectory has to be reproducible bit for bit, and
    % a phase drawn at run time from any RNG - MATLAB's or otherwise - is
    % not a compile-time constant a %#codegen function can carry. They were
    % chosen once, are written here literally, and are not revisited.
    % traj_par(1) is the one free number: an amplitude SCALE, calibrated by
    % verification/traj_check.m so that v_max = 1.26 m/s. y uses the same
    % frequencies with an added quarter-turn-ish phase offset per harmonic,
    % so x and y are not the same signal shifted in time.
    WK  = [0.50, 1.10, 1.90, 2.70];
    PHX = [0.00, 1.30, 2.70, 4.10];
    PHY = [0.80, 2.10, 3.50, 5.60];
    AMPW = [1/0.50, 1/1.10, 1/1.90, 1/2.70];   % flattens each term's velocity peak
    c = traj_par(1);
    [px, vx, ~]    = multisine_axis(t,  WK, PHX, AMPW, c);
    [py, vy, ~]    = multisine_axis(t,  WK, PHY, AMPW, c);
    [~,  ~,  axp]  = multisine_axis(tp, WK, PHX, AMPW, c);
    [~,  ~,  ayp]  = multisine_axis(tp, WK, PHY, AMPW, c);
    gamma_d = [px; py; z0];
    nu_d    = [vx; vy; 0];
    acc_d   = [axp; ayp; 0];

otherwise
    % An unrecognised traj_type is a configuration error, not hover: falling
    % through to hover would make a typo in traj_type invisible - the vehicle
    % would still fly, just not the trajectory anyone asked for. This branch
    % keeps gamma_d/nu_d/acc_d at the zeros() declared above, which for
    % z0 = 0 is at least conspicuously wrong (in the ground) rather than
    % plausibly wrong (a valid-looking hover).
end
end


%% =====================================================================
function [p, v, a] = square_minjerk(t, corners, T, T_h)
%SQUARE_MINJERK  Position/velocity/acceleration on the 4-edge square path.
%
%  corners is 4x2, row k+1 = corner k (k = 0..3, MATLAB 1-indexed rows).
%  Edge k runs from corner k to corner k+1 (mod 4), taking time T, followed
%  by a T_h dwell AT corner k+1 before edge k+1 begins.
p = zeros(2,1); v = zeros(2,1); a = zeros(2,1);

Tcell = T + T_h;
Ttot  = 4*Tcell;
tm    = mod(t, Ttot);
if tm < 0, tm = tm + Ttot; end     % mod() on a negative t in MATLAB Coder
                                    % already returns a nonnegative result for
                                    % a positive Ttot, but this is one line of
                                    % insurance against relying on that.

k   = floor(tm/Tcell);             % 0..3, which edge+dwell slot
if k > 3, k = 3; end               % guards the tm == Ttot boundary sample
tl  = tm - k*Tcell;

k0 = mod(k,   4) + 1;              % 1-indexed row of the START corner
k1 = mod(k+1, 4) + 1;              % 1-indexed row of the END corner
p0 = corners(k0,:).';
p1 = corners(k1,:).';

if tl < T
    s  = tl/T;
    s2 = s*s; s3 = s2*s; s4 = s3*s; s5 = s4*s;
    blend  = 10*s3 - 15*s4 + 6*s5;
    dblend = (30*s2 - 60*s3 + 30*s4)/T;
    ddblend = (60*s - 180*s2 + 120*s3)/T^2;
    d = p1 - p0;
    p = p0 + d*blend;
    v = d*dblend;
    a = d*ddblend;
else
    % Dwell: sitting at the corner just reached.
    p = p1;
    v = zeros(2,1);
    a = zeros(2,1);
end
end


%% =====================================================================
function [p, v, a] = multisine_axis(t, wk, phk, ampw, c)
%MULTISINE_AXIS  One axis of the fixed-frequency multi-sine reference.
%
%  p(t) = c * sum_k ampw(k) * sin(wk(k)*t + phk(k))
%
%  wk, phk, ampw are 1x4 - fixed at the call site, never resized, so this
%  stays codegen-legal with no loop bound that depends on run-time data.
p = 0; v = 0; a = 0;
for k = 1:4
    ph = wk(k)*t + phk(k);
    p = p + c*ampw(k)*sin(ph);
    v = v + c*ampw(k)*wk(k)*cos(ph);
    a = a - c*ampw(k)*wk(k)^2*sin(ph);
end
end
